simulink model "Manual_BCM_Integrated_2020b"  (R2020b)
settings: Solver=VariableStepAuto  StartTime=0.0  StopTime=inf  RelTol=1e-3
undefined symbols (not defined in the file): RES, SET
settings Model: EnablePacing=on  PacingRate=2  Creator=99003729  LastModifiedBy=99003729

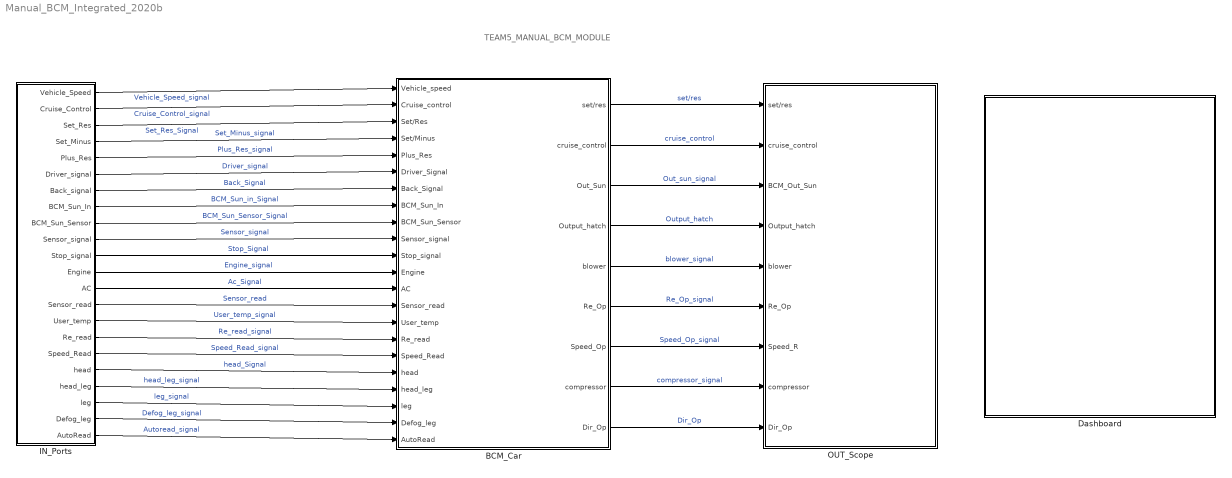
== system Manual_BCM_Integrated_2020b ==
  note: TEAM5_MANUAL_BCM_MODULE
  BCM_Car : Subsystem
  Dashboard : Subsystem
  IN_Ports : Subsystem
  OUT_Scope : Subsystem
  wires:
  IN_Ports/1(Vehicle_Speed) -> BCM_Car/1(Vehicle_speed)  "Vehicle_Speed_signal"
  IN_Ports/2(Cruise_Control) -> BCM_Car/2(Cruise_control)  "Cruise_Control_signal"
  IN_Ports/3(Set_Res) -> BCM_Car/3(Set/Res)  "Set_Res_Signal"
  IN_Ports/4(Set_Minus) -> BCM_Car/4(Set/Minus)  "Set_Minus_signal"
  IN_Ports/5(Plus_Res) -> BCM_Car/5(Plus_Res)  "Plus_Res_signal"
  BCM_Car/1(set/res) -> OUT_Scope/1(set/res)  "set/res"
  BCM_Car/2(cruise_control) -> OUT_Scope/2(cruise_control)  "cruise_control"
  IN_Ports/6(Driver_signal) -> BCM_Car/6(Driver_Signal)  "Driver_signal"
  IN_Ports/7(Back_signal) -> BCM_Car/7(Back_Signal)  "Back_Signal"
  IN_Ports/8(BCM_Sun_In) -> BCM_Car/8(BCM_Sun_In)  "BCM_Sun_in_Signal"
  IN_Ports/9(BCM_Sun_Sensor) -> BCM_Car/9(BCM_Sun_Sensor)  "BCM_Sun_Sensor_Signal"
  BCM_Car/3(Out_Sun) -> OUT_Scope/3(BCM_Out_Sun)  "Out_sun_signal"
  BCM_Car/4(Output_hatch) -> OUT_Scope/4(Output_hatch)  "Output_hatch"
  IN_Ports/10(Sensor_signal) -> BCM_Car/10(Sensor_signal)  "Sensor_signal"
  IN_Ports/11(Stop_signal) -> BCM_Car/11(Stop_signal)  "Stop_Signal"
  IN_Ports/12(Engine) -> BCM_Car/12(Engine)  "Engine_signal"
  IN_Ports/13(AC) -> BCM_Car/13(AC)  "Ac_Signal"
  IN_Ports/14(Sensor_read) -> BCM_Car/14(Sensor_read)  "Sensor_read"
  IN_Ports/15(User_temp) -> BCM_Car/15(User_temp)  "User_temp_signal"
  IN_Ports/16(Re_read) -> BCM_Car/16(Re_read)  "Re_read_signal"
  IN_Ports/17(Speed_Read) -> BCM_Car/17(Speed_Read)  "Speed_Read_signal"
  IN_Ports/18(head) -> BCM_Car/18(head)  "head_Signal"
  IN_Ports/19(head_leg) -> BCM_Car/19(head_leg)  "head_leg_signal"
  IN_Ports/20(leg) -> BCM_Car/20(leg)  "leg_signal"
  IN_Ports/21(Defog_leg) -> BCM_Car/21(Defog_leg)  "Defog_leg_signal"
  IN_Ports/22(AutoRead) -> BCM_Car/22(AutoRead)  "Autoread_signal"
  BCM_Car/5(blower) -> OUT_Scope/5(blower)  "blower_signal"
  BCM_Car/6(Re_Op) -> OUT_Scope/6(Re_Op)  "Re_Op_signal"
  BCM_Car/7(Speed_Op) -> OUT_Scope/7(Speed_R)  "Speed_Op_signal"
  BCM_Car/8(compressor) -> OUT_Scope/8(compressor)  "compressor_signal"
  BCM_Car/9(Dir_Op) -> OUT_Scope/9(Dir_Op)  "Dir_Op"

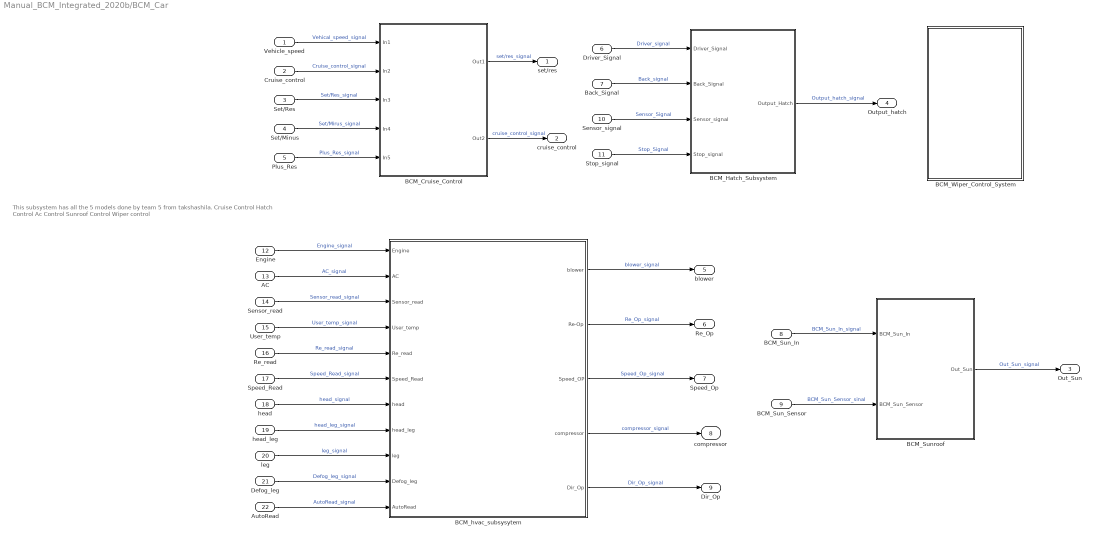
== system Manual_BCM_Integrated_2020b/BCM_Car ==
  note: This subsystem has all the 5 models done by team 5 from takshashila.
      | Cruise Control
      | Hatch Control
      | Ac Control
      | Sunroof Control
      | Wiper control
  Vehicle_speed : Inport
  Cruise_control : Inport  Port=2
  Set/Res : Inport  Port=3
  Set/Minus : Inport  Port=4
  Plus_Res : Inport  Port=5
  Driver_Signal : Inport  Port=6
  Back_Signal : Inport  Port=7
  BCM_Sun_In : Inport  Port=8
  BCM_Sun_Sensor : Inport  Port=9
  Sensor_signal : Inport  Port=10
  Stop_signal : Inport  Port=11
  Engine : Inport  Port=12
  AC : Inport  Port=13
  Sensor_read : Inport  Port=14
  User_temp : Inport  Port=15
  Re_read : Inport  Port=16
  Speed_Read : Inport  Port=17
  head : Inport  Port=18
  head_leg : Inport  Port=19
  leg : Inport  Port=20
  Defog_leg : Inport  Port=21
  AutoRead : Inport  Port=22
  BCM_Cruise_Control : Subsystem
  BCM_Hatch_Subsystem : Subsystem
  BCM_Sunroof : Subsystem
  BCM_Wiper_Control_System : Subsystem
  BCM_hvac_subsysytem : Subsystem
  set/res : Outport
  cruise_control : Outport  Port=2
  Out_Sun : Outport  Port=3
  Output_hatch : Outport  Port=4
  blower : Outport  Port=5
  Re_Op : Outport  Port=6
  Speed_Op : Outport  Port=7
  compressor : Outport  Port=8
  Dir_Op : Outport  Port=9
  wires:
  Vehicle_speed/1 -> BCM_Cruise_Control/1(In1)  "Vehical_speed_signal"
  Cruise_control/1 -> BCM_Cruise_Control/2(In2)  "Cruise_control_signal"
  Set/Res/1 -> BCM_Cruise_Control/3(In3)  "Set/Res_signal"
  Set/Minus/1 -> BCM_Cruise_Control/4(In4)  "Set/Mirus_signal"
  Plus_Res/1 -> BCM_Cruise_Control/5(In5)  "Plus_Res_signal"
  BCM_Cruise_Control/1(Out1) -> set/res/1  "set/res_signal"
  BCM_Cruise_Control/2(Out2) -> cruise_control/1  "cruise_control_signal"
  Driver_Signal/1 -> BCM_Hatch_Subsystem/1(Driver_Signal)  "Driver_signal"
  Back_Signal/1 -> BCM_Hatch_Subsystem/2(Back_Signal)  "Back_signal"
  BCM_Hatch_Subsystem/1(Output_Hatch) -> Output_hatch/1  "Output_hatch_signal"
  BCM_Sun_In/1 -> BCM_Sunroof/1(BCM_Sun_In)  "BCM_Sun_In_signal"
  BCM_Sun_Sensor/1 -> BCM_Sunroof/2(BCM_Sun_Sensor)  "BCM_Sun_Sensor_sinal"
  BCM_Sunroof/1(Out_Sun) -> Out_Sun/1  "Out_Sun_signal"
  Sensor_signal/1 -> BCM_Hatch_Subsystem/3(Sensor_signal)  "Sensor_Signal"
  Stop_signal/1 -> BCM_Hatch_Subsystem/4(Stop_signal)  "Stop_Signal"
  Engine/1 -> BCM_hvac_subsysytem/1(Engine)  "Engine_signal"
  AC/1 -> BCM_hvac_subsysytem/2(AC)  "AC_signal"
  Sensor_read/1 -> BCM_hvac_subsysytem/3(Sensor_read)  "Sensor_read_signal"
  User_temp/1 -> BCM_hvac_subsysytem/4(User_temp)  "User_temp_signal"
  Re_read/1 -> BCM_hvac_subsysytem/5(Re_read)  "Re_read_signal"
  Speed_Read/1 -> BCM_hvac_subsysytem/6(Speed_Read)  "Speed_Read_signal"
  head/1 -> BCM_hvac_subsysytem/7(head)  "head_signal"
  head_leg/1 -> BCM_hvac_subsysytem/8(head_leg)  "head_leg_signal"
  leg/1 -> BCM_hvac_subsysytem/9(leg)  "leg_signal"
  Defog_leg/1 -> BCM_hvac_subsysytem/10(Defog_leg)  "Defog_leg_signal"
  AutoRead/1 -> BCM_hvac_subsysytem/11(AutoRead)  "AutoRead_signal"
  BCM_hvac_subsysytem/1(blower) -> blower/1  "blower_signal"
  BCM_hvac_subsysytem/2(Re-Op) -> Re_Op/1  "Re_Op_signal"
  BCM_hvac_subsysytem/3(Speed_OP) -> Speed_Op/1  "Speed_Op_signal"
  BCM_hvac_subsysytem/4(compressor) -> compressor/1  "compressor_signal"
  BCM_hvac_subsysytem/5(Dir_Op) -> Dir_Op/1  "Dir_Op_signal"

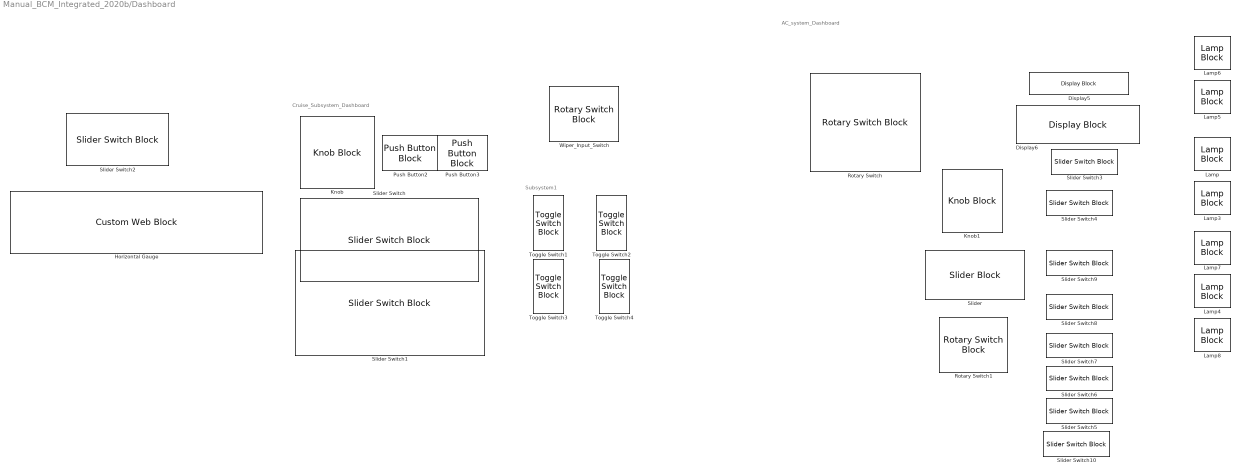
== system Manual_BCM_Integrated_2020b/Dashboard ==
  note: Cruise_Subsystem_Dashboard
  note: Subsystem1
  note: AC_system_Dashboard
  Display5 : DisplayBlock  Format=short  Transparency=1
  Display6 : DisplayBlock  Format=short  Transparency=1
  Horizontal Gauge : CustomWebBlock  ShowInitialText=on  Configuration="{\"components\":[{\"name\":\"LinearScaleComponent\",\"settings\":{\"bounds\":{\"max\":15,\"min\":0,\"tickInterval\":\"auto\"},\"internalTickHeightScaleFactor\":0.5,\"labelColor\":[250,245,199],\"labelFont\":{\"font\":\"Arial\",\"fontSize\":12},\"labelTransparency\":1,\"needleImage\":{\"size\":[21,75],\"src\":\"data:image\\/svg+xml;base64,PHN2ZyB4bWxucz0iaHR0cDovL3d3dy53My5vcmcvMjAwMC9zdmciIHhtbG5zOnhsaW5rPSJodHRwOi8vd3d3LnczLm9yZy8xOTk5L3hsaW5rIiB2aWV3Qm94PSIwIDAgMjEgNzUiPjxkZWZzPjxzdHlsZT4uY2xzLTF7ZmlsbDpub25lO30uY2xzLTJ7aXNvbGF0aW9uOmlzb2xhdGU7fS5jbHMtM3tjbGlwLXBhdGg6dXJsKCNjbGlwLXBhdGgpO30uY2xzLTR7b3BhY2l0eTowLjM7bWl4LWJsZW5kLW1vZGU6bXVsdGlwbHk7fS5jbHMtNXtmaWxsOiNlYjI2Mjk7fTwvc3R5bGU+PGNsaXBQYXRoIGlkPSJjbGlwLXBhdGgiIHRyYW5zZm9y ...(+1928 chars)\",\"srcOrientation\":\"horizontal\"},\"needleOffset\":[0,0.01094391244870041],\"needleSize\":{\"height\":0.7589285714285714,\"width\":0.11960078534031414},\"position\":[0.06986607142857143,0.01995798319327731,0.9641544117647058,0.8],\"scaleColors\":[],\"scaleColorsSize\":0.2,\"showLabels\":1,\"showMinorTicks\":0,\"showSpanLine\":1,\"showTicks\":1,\"tickColor\":[250,245,200],\"tickTransparency\":1,\"valueBarColor\":[23,89,176],\"valueBarOffset\":0,\"valueBarSize\":0.23,\"valueBarTransparency\":1}},{\"name\":\"BackgroundImageComponent\",\"settings\":{\"image\":{\"size\":[380,101],\"src\":\"data:image\\/svg+xml;base64,PHN2ZyB4bWxucz0iaHR0cDovL3d3dy53My5vcmcvMjAwMC9zdmciIHZpZXdCb3g9IjAgMCAzODAgMTAxIj48ZGVmcz48c3R5bGU+LmNscy0xe2ZpbGw6IzAwMmI0Mjt9LmNscy0ye2ZpbGw6IzQyNzA4Mjt9LmNscy0ze2ZpbGw6IzdjYTBiMjt9PC9zdHlsZT48L2RlZnM+PHRpdGxlPmhvcml6b250YWxfZ2F1Z2VfIGJhY2tncm91bmQ8L3RpdGxlPjxnIGlkPSJMYXllcl8yIiBkYXRhLW5hbWU9IkxheWVyIDIiPjxnIGlkPSJMYXllcl8xLTIiIGRhdGEtbmFtZT0iTGF5ZXIgMSI+PHJlY3QgY2xhc3M9ImNscy0xIiB4PSIxMSIgeT0iMTEiIHdpZHRoPSIzNTgiIGhlaWdodD0iNzkiLz48cGF0aCBjbGFzcz0iY2xzLTIiIGQ9Ik04LDhWOTNIMzcyVjhaTTM2OSw5MEgxMVYxMUgzNjlaIi8+PHBhdGggY2xhc3M9ImNscy0zIiBkPSJNMCwwVjEwMUgzODBWMFpNMzcyLDkzSDhWOEgzNzJaIi8+PC9nPjwvZz48L3N2Zz4=\",\"srcOrientation\":\"horizontal\"},\"position\":[0,0,1,1],\"scaleMode\":\"0\"}},{\"name\":\"ForegroundImageComponent\",\"settings\":{\"image\":{\"size\":[0,0],\"src\":\"default\",\"srcOrientation\":[]},\"isForeground\":1,\"position\":[0,0,1,1],\"scaleMode\":\"0\"}}],\"settings\":{\"BindingType\":\"signal\",\"aspectRatio\":3.7777777777777777,\"fixedAspectRatio\":\"on\",\"orientation\":\"horizontal\"},\"type\":\"LinearGauge\"}"
  Knob : KnobBlock
  Knob1 : KnobBlock  ScaleMax=50
  Lamp{,3..8} (7 alike) : LampBlock
  Push Button2 : PushButtonBlock  ButtonText=SET-
  Push Button3 : PushButtonBlock  ButtonText=+RES
  Rotary Switch : RotarySwitchBlock
      settings: Values={{'Off', 'Low', 'Medium', 'High'}, [0 1 2 3]}
  Rotary Switch1 : RotarySwitchBlock
      settings: Values={{'Low', 'Medium', 'High'}, [1 2 3]}
  Slider : SliderBlock  ScaleMax=50
  Slider Switch{,1..10} (11 alike) : SliderSwitchBlock
  Toggle Switch{1..4} (4 alike) : ToggleSwitchBlock
  Wiper_Input_Switch : RotarySwitchBlock
      settings: Values={{'Off', 'Low', 'Medium', 'High', 'Mist'}, [5 1 2 3 4]}

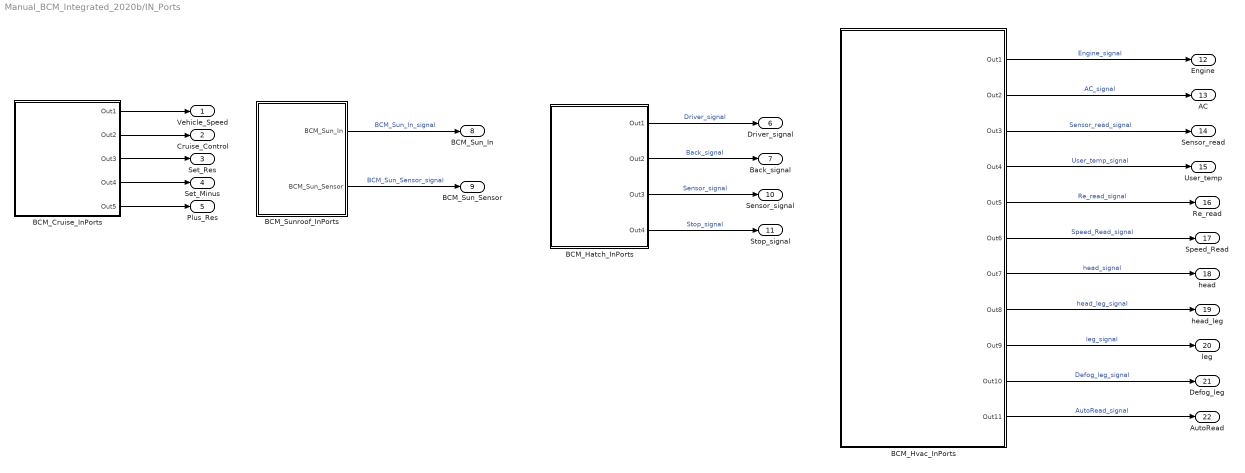
== system Manual_BCM_Integrated_2020b/IN_Ports ==
  BCM_Cruise_InPorts : Subsystem
  BCM_Hatch_InPorts : Subsystem
  BCM_Hvac_InPorts : Subsystem
  BCM_Sunroof_InPorts : Subsystem
  Vehicle_Speed : Outport
  Cruise_Control : Outport  Port=2
  Set_Res : Outport  Port=3
  Set_Minus : Outport  Port=4
  Plus_Res : Outport  Port=5
  Driver_signal : Outport  Port=6
  Back_signal : Outport  Port=7
  BCM_Sun_In : Outport  Port=8
  BCM_Sun_Sensor : Outport  Port=9
  Sensor_signal : Outport  Port=10
  Stop_signal : Outport  Port=11
  Engine : Outport  Port=12
  AC : Outport  Port=13
  Sensor_read : Outport  Port=14
  User_temp : Outport  Port=15
  Re_read : Outport  Port=16
  Speed_Read : Outport  Port=17
  head : Outport  Port=18
  head_leg : Outport  Port=19
  leg : Outport  Port=20
  Defog_leg : Outport  Port=21
  AutoRead : Outport  Port=22
  wires:
  BCM_Cruise_InPorts/1(Out1) -> Vehicle_Speed/1
  BCM_Cruise_InPorts/2(Out2) -> Cruise_Control/1
  BCM_Cruise_InPorts/3(Out3) -> Set_Res/1
  BCM_Cruise_InPorts/4(Out4) -> Set_Minus/1
  BCM_Cruise_InPorts/5(Out5) -> Plus_Res/1
  BCM_Hatch_InPorts/1(Out1) -> Driver_signal/1  "Driver_signal"
  BCM_Hatch_InPorts/2(Out2) -> Back_signal/1  "Back_signal"
  BCM_Sunroof_InPorts/1(BCM_Sun_In) -> BCM_Sun_In/1  "BCM_Sun_In_signal"
  BCM_Sunroof_InPorts/2(BCM_Sun_Sensor) -> BCM_Sun_Sensor/1  "BCM_Sun_Sensor_signal"
  BCM_Hatch_InPorts/3(Out3) -> Sensor_signal/1  "Sensor_signal"
  BCM_Hatch_InPorts/4(Out4) -> Stop_signal/1  "Stop_signal"
  BCM_Hvac_InPorts/1(Out1) -> Engine/1  "Engine_signal"
  BCM_Hvac_InPorts/2(Out2) -> AC/1  "AC_signal"
  BCM_Hvac_InPorts/3(Out3) -> Sensor_read/1  "Sensor_read_signal"
  BCM_Hvac_InPorts/4(Out4) -> User_temp/1  "User_temp_signal"
  BCM_Hvac_InPorts/5(Out5) -> Re_read/1  "Re_read_signal"
  BCM_Hvac_InPorts/6(Out6) -> Speed_Read/1  "Speed_Read_signal"
  BCM_Hvac_InPorts/7(Out7) -> head/1  "head_signal"
  BCM_Hvac_InPorts/8(Out8) -> head_leg/1  "head_leg_signal"
  BCM_Hvac_InPorts/9(Out9) -> leg/1  "leg_signal"
  BCM_Hvac_InPorts/10(Out10) -> Defog_leg/1  "Defog_leg_signal"
  BCM_Hvac_InPorts/11(Out11) -> AutoRead/1  "AutoRead_signal"

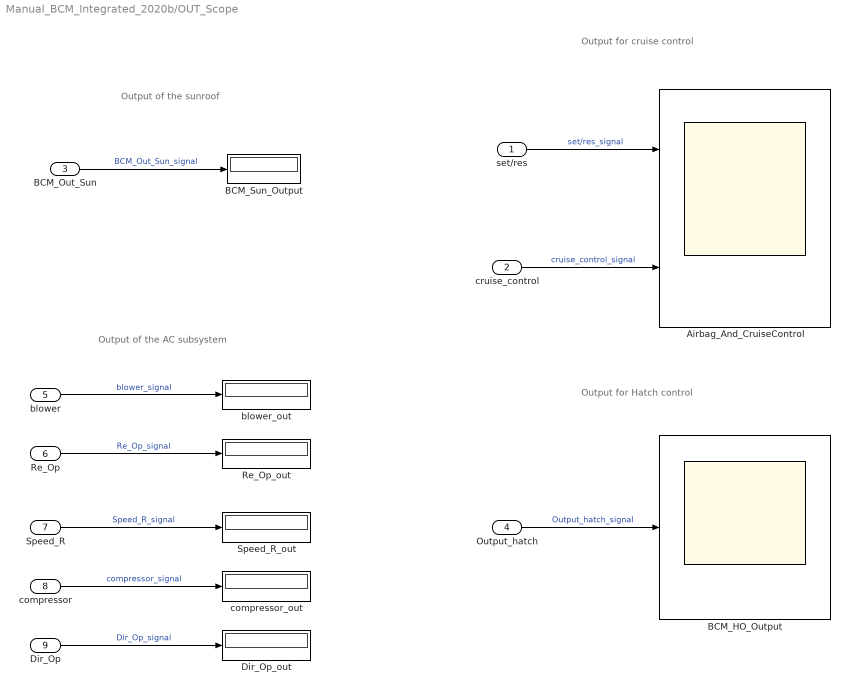
== system Manual_BCM_Integrated_2020b/OUT_Scope ==
  note: Output for cruise control
  note: Output of the sunroof
  note: Output of the AC subsystem
  note: Output for Hatch control
  set/res : Inport
  cruise_control : Inport  Port=2
  BCM_Out_Sun : Inport  Port=3
  Output_hatch : Inport  Port=4
  blower : Inport  Port=5
  Re_Op : Inport  Port=6
  Speed_R : Inport  Port=7
  compressor : Inport  Port=8
  Dir_Op : Inport  Port=9
  Airbag_And_CruiseControl : Scope  NumInputPorts=2
  BCM_HO_Output : Scope
  BCM_Sun_Output : Display
  Dir_Op_out : Display
  Re_Op_out : Display
  Speed_R_out : Display
  blower_out : Display
  compressor_out : Display
  wires:
  set/res/1 -> Airbag_And_CruiseControl/1  "set/res_signal"
  cruise_control/1 -> Airbag_And_CruiseControl/2  "cruise_control_signal"
  BCM_Out_Sun/1 -> BCM_Sun_Output/1  "BCM_Out_Sun_signal"
  Output_hatch/1 -> BCM_HO_Output/1  "Output_hatch_signal"
  blower/1 -> blower_out/1  "blower_signal"
  Re_Op/1 -> Re_Op_out/1  "Re_Op_signal"
  Speed_R/1 -> Speed_R_out/1  "Speed_R_signal"
  compressor/1 -> compressor_out/1  "compressor_signal"
  Dir_Op/1 -> Dir_Op_out/1  "Dir_Op_signal"

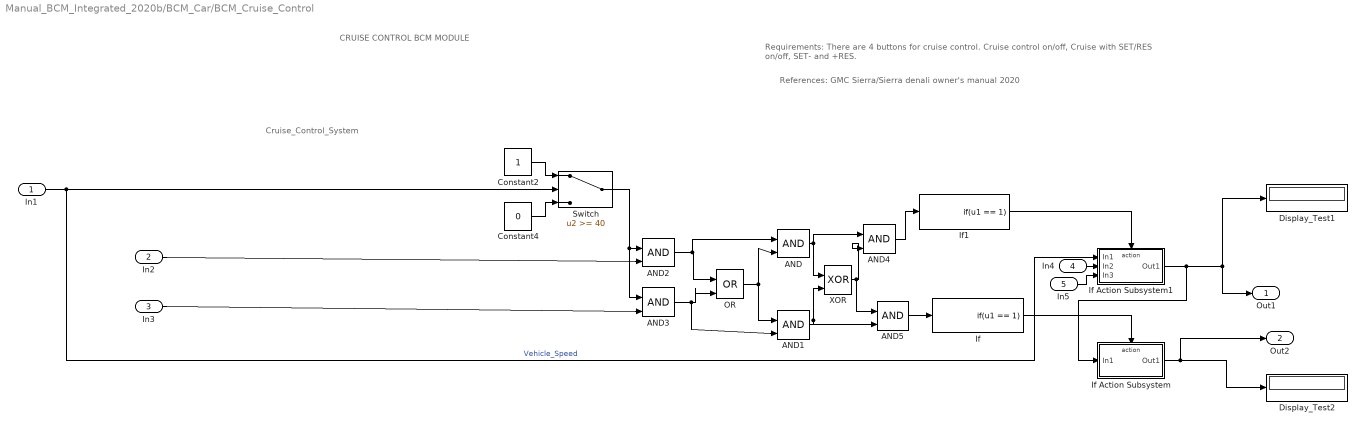
== system Manual_BCM_Integrated_2020b/BCM_Car/BCM_Cruise_Control ==
  note: Cruise_Control_System
  note: CRUISE CONTROL BCM MODULE
  note: References: GMC Sierra/Sierra denali owner's manual 2020
  note: Requirements: There are 4 buttons for cruise control. Cruise control on/off, Cruise with SET/RES on/off, SET- and +RES.
  In1 : Inport
  In2 : Inport  Port=2
  In3 : Inport  Port=3
  In4 : Inport  Port=4
  In5 : Inport  Port=5
  AND{,1..5} (6 alike) : Logic  IconShape=distinctive  AllPortsSameDT=off  OutDataTypeStr=boolean
  Constant2 : Constant
  Constant4 : Constant  Value=0
  Display_Test1 : Display
  Display_Test2 : Display
  If : If  IfExpression=u1 == 1  ShowElse=off
  If Action Subsystem : Subsystem  TreatAsAtomicUnit=on
  If Action Subsystem1 : Subsystem  TreatAsAtomicUnit=on
  If1 : If  IfExpression=u1 == 1  ShowElse=off
  OR : Logic  Operator=OR  IconShape=distinctive  AllPortsSameDT=off  OutDataTypeStr=boolean
  Switch : Switch  Threshold=40
  XOR : Logic  Operator=XOR  IconShape=distinctive  AllPortsSameDT=off  OutDataTypeStr=boolean
  Out1 : Outport
  Out2 : Outport  Port=2
  wires:
  AND5/1 -> If/1
  If1/1 -> If Action Subsystem1/Action
  If/1 -> If Action Subsystem/Action
  If Action Subsystem/1(Out1) -> Out2/1, Display_Test2/1
  AND/1 -> AND4/1, XOR/1
  XOR/1 -> AND5/1, AND4/2
  In1/1 -> Switch/2, If Action Subsystem1/1(In1)  "Vehicle_Speed"
  OR/1 -> AND1/1, AND/2
  AND2/1 -> AND/1, OR/1
  In2/1 -> AND2/2
  Constant4/1 -> Switch/3
  AND3/1 -> AND1/2, OR/2
  AND1/1 -> XOR/2, AND5/2
  Switch/1 -> AND3/1, AND2/1
  Constant2/1 -> Switch/1
  AND4/1 -> If1/1
  If Action Subsystem1/1(Out1) -> If Action Subsystem/1(In1), Out1/1, Display_Test1/1
  In3/1 -> AND3/2
  In4/1 -> If Action Subsystem1/2(In2)
  In5/1 -> If Action Subsystem1/3(In3)

== system Manual_BCM_Integrated_2020b/BCM_Car/BCM_Hatch_Subsystem ==
  Driver_Signal : Inport
  Back_Signal : Inport  Port=2
  Sensor_signal : Inport  Port=3
  Stop_signal : Inport  Port=4
  BCM_HO_Controller : Subsystem
  Output_Hatch : Outport
  wires:
  Driver_Signal/1 -> BCM_HO_Controller/1(Driver_Signal)  "Driver_Signal"
  Back_Signal/1 -> BCM_HO_Controller/2(Back_Signal)  "Back_Signal"
  Sensor_signal/1 -> BCM_HO_Controller/3(Sensor_signal)  "Sensor_signal"
  Stop_signal/1 -> BCM_HO_Controller/4(Stop_signal)  "Stop_signal"
  BCM_HO_Controller/1(Out1) -> Output_Hatch/1  "Output_Hatch_signal"

== system Manual_BCM_Integrated_2020b/BCM_Car/BCM_Sunroof ==
  note: Functioning of sunroof
  note: Requierments
      | u - sunroof input
      | v - sensor input
  BCM_Sun_In : Inport
  BCM_Sun_Sensor : Inport  Port=2
  Function_Sun : MATLAB Function  TreatAsAtomicUnit=on
  Out_Sun : Outport
  wires:
  BCM_Sun_Sensor/1 -> Function_Sun/2(v)  "Sun_sensor_signal"
  BCM_Sun_In/1 -> Function_Sun/1(u)  "Sun_In_signal"
  Function_Sun/1(y) -> Out_Sun/1  "BCM_Out_Sun"

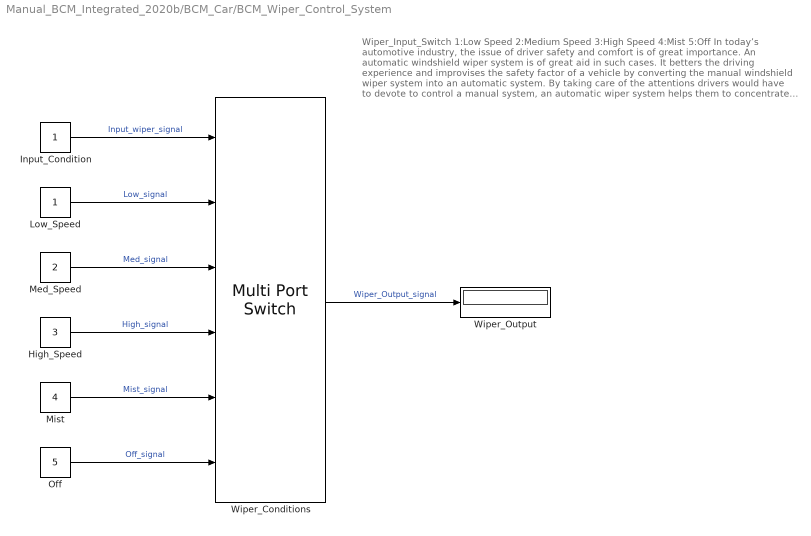
== system Manual_BCM_Integrated_2020b/BCM_Car/BCM_Wiper_Control_System ==
  note: Wiper_Input_Switch
      | 1:Low Speed
      | 2:Medium Speed
      | 3:High Speed
      | 4:Mist
      | 5:Off
      | In today’s automotive industry, the issue of driver safety and comfort is of great importance. An automatic windshield wiper system is of great aid in such cases. It betters the driving experience and improvises the safety factor of a vehicle by converting the manual windshield wiper system into an automatic system. By taking care of the attentions drivers would have to devote to control a manual system, an automatic wiper system helps them to concentrate more on driving safely. Although, few automated windshield wiper systems are available in the automotive market, they are very costly and not very effective.
  High_Speed : Constant  Value=3
  Input_Condition : Constant
  Low_Speed : Constant
  Med_Speed : Constant  Value=2
  Mist : Constant  Value=4
  Off : Constant  Value=5
  Wiper_Conditions : MultiPortSwitch  Inputs=5
  Wiper_Output : Display
  wires:
  Wiper_Conditions/1 -> Wiper_Output/1  "Wiper_Output_signal"
  Med_Speed/1 -> Wiper_Conditions/3  "Med_signal"
  Off/1 -> Wiper_Conditions/6  "Off_signal"
  Mist/1 -> Wiper_Conditions/5  "Mist_signal"
  Input_Condition/1 -> Wiper_Conditions/1  "Input_wiper_signal"
  High_Speed/1 -> Wiper_Conditions/4  "High_signal"
  Low_Speed/1 -> Wiper_Conditions/2  "Low_signal"

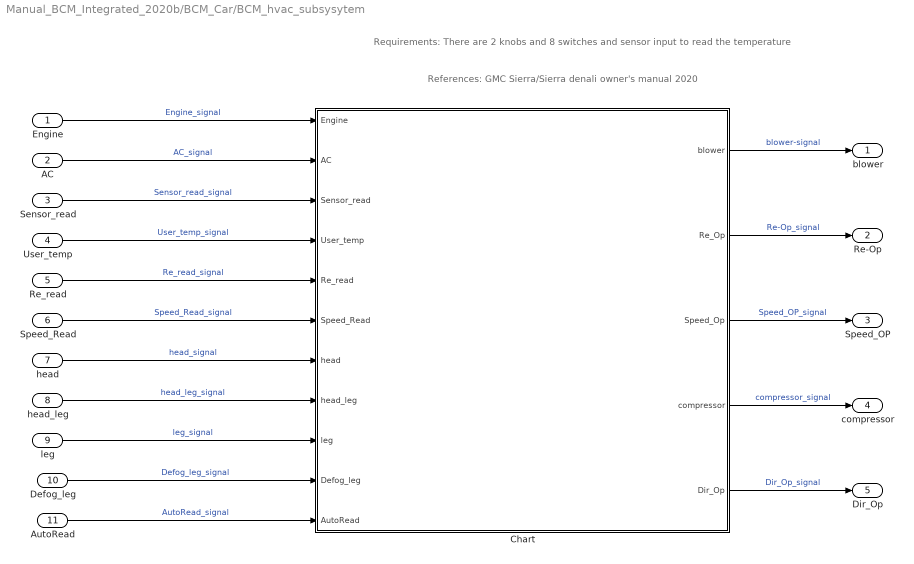
== system Manual_BCM_Integrated_2020b/BCM_Car/BCM_hvac_subsysytem ==
  note: References: GMC Sierra/Sierra denali owner's manual 2020
  note: Requirements: There are 2 knobs and 8 switches and sensor input to read the temperature
  Engine : Inport
  AC : Inport  Port=2
  Sensor_read : Inport  Port=3
  User_temp : Inport  Port=4
  Re_read : Inport  Port=5
  Speed_Read : Inport  Port=6
  head : Inport  Port=7
  head_leg : Inport  Port=8
  leg : Inport  Port=9
  Defog_leg : Inport  Port=10
  AutoRead : Inport  Port=11
  Chart : Stateflow chart  TreatAsAtomicUnit=on
  blower : Outport
  Re-Op : Outport  Port=2
  Speed_OP : Outport  Port=3
  compressor : Outport  Port=4
  Dir_Op : Outport  Port=5
  wires:
  Engine/1 -> Chart/1(Engine)  "Engine_signal"
  AC/1 -> Chart/2(AC)  "AC_signal"
  Sensor_read/1 -> Chart/3(Sensor_read)  "Sensor_read_signal"
  User_temp/1 -> Chart/4(User_temp)  "User_temp_signal"
  Re_read/1 -> Chart/5(Re_read)  "Re_read_signal"
  Speed_Read/1 -> Chart/6(Speed_Read)  "Speed_Read_signal"
  head/1 -> Chart/7(head)  "head_signal"
  head_leg/1 -> Chart/8(head_leg)  "head_leg_signal"
  leg/1 -> Chart/9(leg)  "leg_signal"
  Defog_leg/1 -> Chart/10(Defog_leg)  "Defog_leg_signal"
  AutoRead/1 -> Chart/11(AutoRead)  "AutoRead_signal"
  Chart/1(blower) -> blower/1  "blower-signal"
  Chart/2(Re_Op) -> Re-Op/1  "Re-Op_signal"
  Chart/3(Speed_Op) -> Speed_OP/1  "Speed_OP_signal"
  Chart/4(compressor) -> compressor/1  "compressor_signal"
  Chart/5(Dir_Op) -> Dir_Op/1  "Dir_Op_signal"

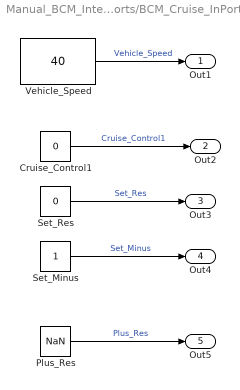
== system Manual_BCM_Integrated_2020b/IN_Ports/BCM_Cruise_InPorts ==
  Cruise_Control1 : Constant  Value=0
  Plus_Res : Constant  Value=NaN
  Set_Minus : Constant
  Set_Res : Constant  Value=0
  Vehicle_Speed : Constant  Value=40
  Out1 : Outport
  Out2 : Outport  Port=2
  Out3 : Outport  Port=3
  Out4 : Outport  Port=4
  Out5 : Outport  Port=5
  wires:
  Vehicle_Speed/1 -> Out1/1  "Vehicle_Speed"
  Cruise_Control1/1 -> Out2/1  "Cruise_Control1"
  Set_Res/1 -> Out3/1  "Set_Res"
  Set_Minus/1 -> Out4/1  "Set_Minus"
  Plus_Res/1 -> Out5/1  "Plus_Res"

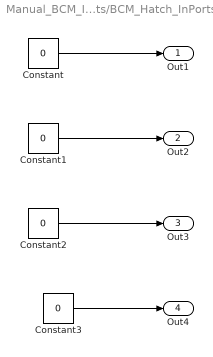
== system Manual_BCM_Integrated_2020b/IN_Ports/BCM_Hatch_InPorts ==
  Constant{,1..3} (4 alike) : Constant  Value=0
  Out1 : Outport
  Out2 : Outport  Port=2
  Out3 : Outport  Port=3
  Out4 : Outport  Port=4
  wires:
  Constant/1 -> Out1/1
  Constant1/1 -> Out2/1
  Constant3/1 -> Out4/1
  Constant2/1 -> Out3/1

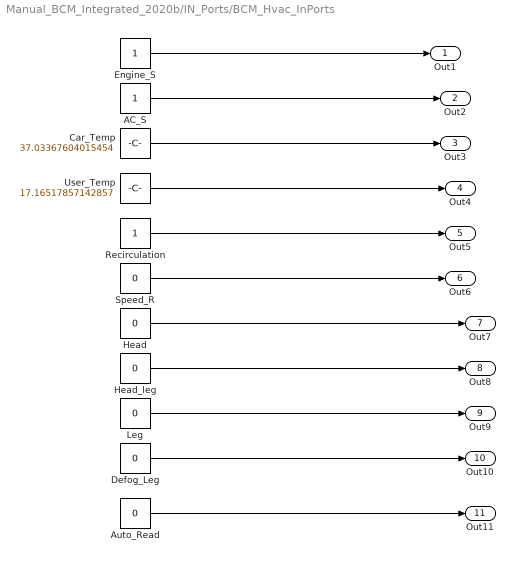
== system Manual_BCM_Integrated_2020b/IN_Ports/BCM_Hvac_InPorts ==
  AC_S : Constant
  Auto_Read : Constant  Value=0
  Car_Temp : Constant  Value=37.03367604015454
  Defog_Leg : Constant  Value=0
  Engine_S : Constant
  Head : Constant  Value=0
  Head_leg : Constant  Value=0
  Leg : Constant  Value=0
  Recirculation : Constant
  Speed_R : Constant  Value=0
  User_Temp : Constant  Value=17.16517857142857
  Out1 : Outport
  Out2 : Outport  Port=2
  Out3 : Outport  Port=3
  Out4 : Outport  Port=4
  Out5 : Outport  Port=5
  Out6 : Outport  Port=6
  Out7 : Outport  Port=7
  Out8 : Outport  Port=8
  Out9 : Outport  Port=9
  Out10 : Outport  Port=10
  Out11 : Outport  Port=11
  wires:
  Engine_S/1 -> Out1/1
  Auto_Read/1 -> Out11/1
  Defog_Leg/1 -> Out10/1
  Car_Temp/1 -> Out3/1
  AC_S/1 -> Out2/1
  Recirculation/1 -> Out5/1
  Head/1 -> Out7/1
  User_Temp/1 -> Out4/1
  Leg/1 -> Out9/1
  Speed_R/1 -> Out6/1
  Head_leg/1 -> Out8/1

== system Manual_BCM_Integrated_2020b/IN_Ports/BCM_Sunroof_InPorts ==
  note: Inputs of the sunroof system
  note: Sunroof_Inputs
      | 0 - off
      | 1 - siglepress
      | 2 - fullpress
      | Sensor_For_Object
      | 0 - no object
      | 1 - object
  BCM_Sun_Inp : Constant  Value=0
  BCM_Sun_Sens : Constant  Value=0
  BCM_Sun_In : Outport
  BCM_Sun_Sensor : Outport  Port=2
  wires:
  BCM_Sun_Sens/1 -> BCM_Sun_Sensor/1  "BCM_Sun_Sensor_signal"
  BCM_Sun_Inp/1 -> BCM_Sun_In/1  "BCM_Sun_In_signal"

== system Manual_BCM_Integrated_2020b/BCM_Car/BCM_Cruise_Control/If Action Subsystem ==
  In1 : Inport
  Action Port : ActionPort  ActionPortLabel=if(u1 == 1)
  Out1 : Outport
  wires:
  In1/1 -> Out1/1

== system Manual_BCM_Integrated_2020b/BCM_Car/BCM_Cruise_Control/If Action Subsystem1 ==
  In1 : Inport
  In2 : Inport  Port=2
  In3 : Inport  Port=3
  Action Port : ActionPort  ActionPortLabel=if(u1 == 1)
  Add : Sum
  Chart : Stateflow chart  TreatAsAtomicUnit=on
  Out1 : Outport
  wires:
  Add/1 -> Out1/1
  Chart/1(data) -> Add/1
  In1/1 -> Add/2
  In3/1 -> Chart/2(inc)
  In2/1 -> Chart/1(dec)

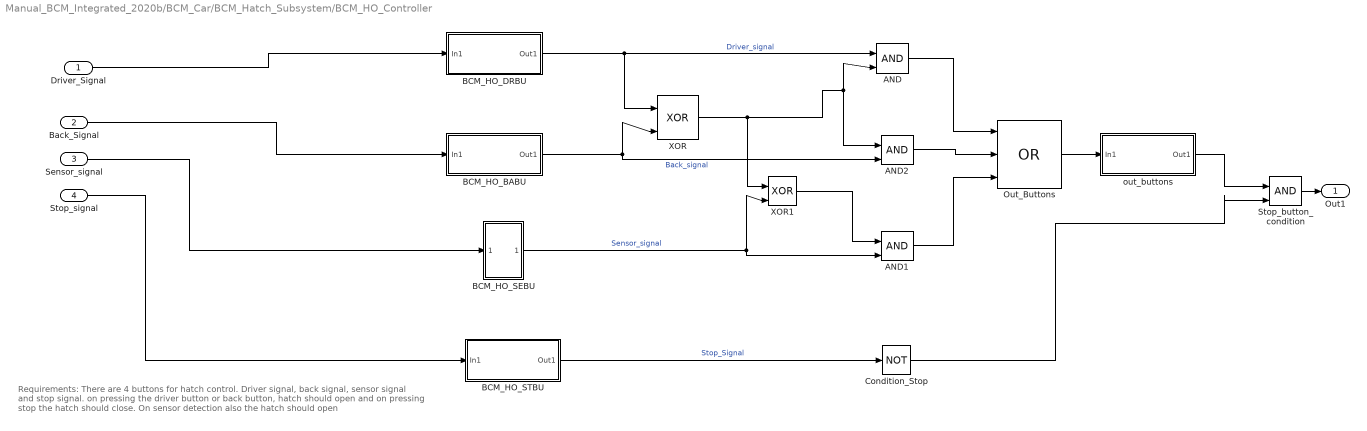
== system Manual_BCM_Integrated_2020b/BCM_Car/BCM_Hatch_Subsystem/BCM_HO_Controller ==
  note: Requirements: There are 4 buttons for hatch control. Driver signal, back signal, sensor signal and stop signal. on pressing the driver button or back button, hatch should open and on pressing stop the hatch should close. On sensor detection also the hatch should open
  Driver_Signal : Inport
  Back_Signal : Inport  Port=2
  Sensor_signal : Inport  Port=3
  Stop_signal : Inport  Port=4
  AND : Logic  IconShape=distinctive  AllPortsSameDT=off  OutDataTypeStr=boolean
  AND1 : Logic  IconShape=distinctive  AllPortsSameDT=off  OutDataTypeStr=boolean
  AND2 : Logic  IconShape=distinctive  AllPortsSameDT=off  OutDataTypeStr=boolean
  BCM_HO_BABU : Subsystem
  BCM_HO_DRBU : Subsystem
  BCM_HO_SEBU : Subsystem
  BCM_HO_STBU : Subsystem
  Condition_Stop : Logic  Operator=NOT  IconShape=distinctive  AllPortsSameDT=off  OutDataTypeStr=boolean
  Out_Buttons : Logic  Operator=OR  Inputs=3  IconShape=distinctive  AllPortsSameDT=off  OutDataTypeStr=boolean
  Stop_button_condition : Logic  IconShape=distinctive  AllPortsSameDT=off  OutDataTypeStr=boolean
  XOR : Logic  Operator=XOR  IconShape=distinctive  AllPortsSameDT=off  OutDataTypeStr=boolean
  XOR1 : Logic  Operator=XOR  IconShape=distinctive  AllPortsSameDT=off  OutDataTypeStr=boolean
  out_buttons : Subsystem
  Out1 : Outport
  wires:
  BCM_HO_SEBU/1(Out1) -> XOR1/2, AND1/2  "Sensor_signal"
  Stop_signal/1 -> BCM_HO_STBU/1(In1)
  XOR/1 -> XOR1/1, AND2/1, AND/2
  XOR1/1 -> AND1/1
  AND2/1 -> Out_Buttons/2
  Condition_Stop/1 -> Stop_button_condition/2
  BCM_HO_BABU/1(Out1) -> XOR/2, AND2/2  "Back_signal"
  AND/1 -> Out_Buttons/1
  Out_Buttons/1 -> out_buttons/1(In1)
  AND1/1 -> Out_Buttons/3
  BCM_HO_STBU/1(Out1) -> Condition_Stop/1  "Stop_Signal"
  out_buttons/1(Out1) -> Stop_button_condition/1
  BCM_HO_DRBU/1(Out1) -> AND/1, XOR/1  "Driver_signal"
  Sensor_signal/1 -> BCM_HO_SEBU/1(In1)
  Driver_Signal/1 -> BCM_HO_DRBU/1(In1)
  Back_Signal/1 -> BCM_HO_BABU/1(In1)
  Stop_button_condition/1 -> Out1/1

== system Manual_BCM_Integrated_2020b/BCM_Car/BCM_Hatch_Subsystem/BCM_HO_Controller/BCM_HO_BABU ==
  In1 : Inport
  Out1 : Outport
  wires:
  In1/1 -> Out1/1

== system Manual_BCM_Integrated_2020b/BCM_Car/BCM_Hatch_Subsystem/BCM_HO_Controller/BCM_HO_DRBU ==
  In1 : Inport
  Out1 : Outport
  wires:
  In1/1 -> Out1/1

== system Manual_BCM_Integrated_2020b/BCM_Car/BCM_Hatch_Subsystem/BCM_HO_Controller/BCM_HO_SEBU ==
  In1 : Inport
  Constant1 : Constant
  Constant2 : Constant  Value=0
  Saturation : Saturate  UpperLimit=3.6  LowerLimit=0
  Subsystem1 : Subsystem
  Switch : Switch  Criteria=u2 > Threshold  Threshold=2.3
  Out1 : Outport
  wires:
  In1/1 -> Subsystem1/1(In1)
  Saturation/1 -> Switch/2
  Constant1/1 -> Switch/1
  Constant2/1 -> Switch/3
  Switch/1 -> Out1/1
  Subsystem1/1(Out1) -> Saturation/1

== system Manual_BCM_Integrated_2020b/BCM_Car/BCM_Hatch_Subsystem/BCM_HO_Controller/BCM_HO_STBU ==
  In1 : Inport
  Out1 : Outport
  wires:
  In1/1 -> Out1/1

== system Manual_BCM_Integrated_2020b/BCM_Car/BCM_Hatch_Subsystem/BCM_HO_Controller/out_buttons ==
  In1 : Inport
  Out1 : Outport
  wires:
  In1/1 -> Out1/1

== system Manual_BCM_Integrated_2020b/BCM_Car/BCM_Hatch_Subsystem/BCM_HO_Controller/BCM_HO_SEBU/Subsystem1 ==
  In1 : Inport
  Out1 : Outport
  wires:
  In1/1 -> Out1/1

== matlab function Manual_BCM_Integrated_2020b/BCM_Car/BCM_Sunroof/Function_Sun ==
  data: u input; y output; v input
function y = fcn(u,v)
if u == 1
    for i = 1:5
        y = u * i;
    end
elseif u == 2
    for i = 1:5
        y = u * i;
    end
elseif u == 3
    for i = 1:5
        y = u * i;
    end
else
    y = u;
end
if v == 1 && u ~= 0
   y = 15;
end

== stateflow chart Manual_BCM_Integrated_2020b/BCM_Car/BCM_hvac_subsysytem/Chart ==
  state AC_ON
    en:
    blower= 1;
    if Re_read==1
    Re_Op = 1;
    else
    Re_Op = 0;
    end
    (default) -> (junction 28) : % Blower_speed
    (junction 28) -> (junction 29) [order 1] : [Speed_Read == 2]
    (junction 28) -> (junction 30) [order 2]
    (junction 29) -> (junction 34) : {Speed_Op = 2;}
    (junction 30) -> (junction 31) [order 1] : [Speed_Read == 3]
    (junction 30) -> (junction 32) [order 2] : {Speed_Op =1;}
    (junction 31) -> (junction 33) : {Speed_Op = 3;}
    (junction 33) -> (junction 32)
    (junction 34) -> (junction 33)
    (junction 32) -> (junction 35)
  state Compressor_cond
    en:
    compressor = 1;
  state HVAC_OFF
    en:
    blower=0;
    compressor=0;
  state Compressor_cond1
    en:
    compressor = 0;
  state Auto_cond
    (default) -> (junction 67) : % Auto_cond
    (junction 67) -> (junction 68) [order 1] : [head == 1 ]
    (junction 67) -> (junction 69) [order 2]
    (junction 68) -> (junction 76) : {Dir_Op = 1;}
    (junction 69) -> (junction 70) [order 1] : [leg == 1]
    (junction 69) -> (junction 71) [order 2]
    (junction 70) -> (junction 75) : {Dir_Op = 2;}
    (junction 71) -> (junction 72) [order 1] : [head_leg == 1]
    (junction 71) -> (junction 73) [order 2]
    (junction 72) -> (junction 74) : {Dir_Op = 3;}
    (junction 73) -> (junction 79) [order 1] : [Defog_leg == 1]
    (junction 73) -> (junction 77) [order 2] : {Dir_Op = 0;}
    (junction 79) -> (junction 78) : {Dir_Op = 4;}
    (junction 78) -> (junction 77)
    (junction 74) -> (junction 78)
    (junction 75) -> (junction 74)
    (junction 76) -> (junction 75)
  AC_ON -> Compressor_cond [order 2] : [User_temp < Sensor_read && compressor ==0 ]
  (default) -> HVAC_OFF
  Compressor_cond -> AC_ON : after(0.5,usec)
  HVAC_OFF -> AC_ON : [Engine == 1 && AC ==1]
  AC_ON -> HVAC_OFF [order 1] : [Engine ==0 || AC == 0]
  AC_ON -> Compressor_cond1 [order 3] : [User_temp >= Sensor_read && compressor ==1]
  Compressor_cond1 -> AC_ON : after(0.5,usec)
  Auto_cond -> AC_ON : after(0.5,usec)
  AC_ON -> Auto_cond [order 4] : [AutoRead==1|| head ==1 || head_leg ==1 || leg == 1 || Defog_leg == 1]
  data: Engine input; AC input; blower output; Sensor_read input; User_temp input; Re_read input; Re_Op output; Speed_Op output; Speed_Read input; compressor output; head input; head_leg input; leg input; Defog_leg input; Dir_Op output; AutoRead input

== stateflow chart Manual_BCM_Integrated_2020b/BCM_Car/BCM_Cruise_Control/If Action Subsystem1/Chart ==
  state main
    during:
    if inc==1
    data=data+1;
    end
    if dec==1
    data=data-1;
    end
  (default) -> main
  data: dec input; inc input; data output =0
